simulink model "part2"  (R2017b)
settings: Solver=VariableStepAuto  StartTime=0.0  StopTime=5  MaxStep=0.001  RelTol=1e-3
settings Model: Creator=ras19  LastModifiedBy=drone
settings CodeAppCC: StateflowObjectComments=on

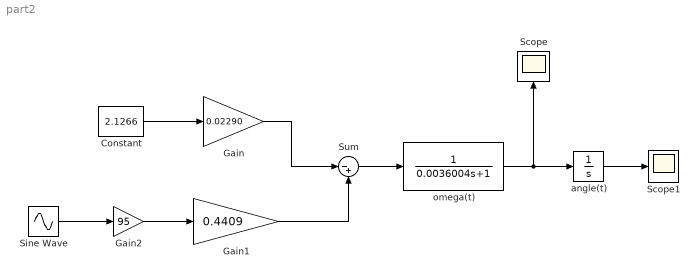
== system part2 ==
  Constant : Constant  Value=2.1266
  Gain : Gain  Gain=0.02290
  Gain1 : Gain  Gain=0.4409
  Gain2 : Gain  Gain=95
  Scope : Scope
  Scope1 : Scope
  Sine Wave : Sin  Amplitude=0.5233  Frequency=7.5  SampleTime=0
  Sum : Sum  Inputs=|-+
  angle(t) : Integrator
  omega(t) : TransferFcn  Denominator=[0.0036004 1]
  wires:
  Constant/1 -> Gain/1
  Gain/1 -> Sum/1
  Gain1/1 -> Sum/2
  Sum/1 -> omega(t)/1
  omega(t)/1 -> angle(t)/1, Scope/1
  angle(t)/1 -> Scope1/1
  Gain2/1 -> Gain1/1
  Sine Wave/1 -> Gain2/1
